simulink model "Switch_block"  (R2021a)
settings: Solver=VariableStepAuto  StartTime=0.0  StopTime=10.0  RelTol=1e-3
settings Model: Creator=HP  LastModifiedBy=HP

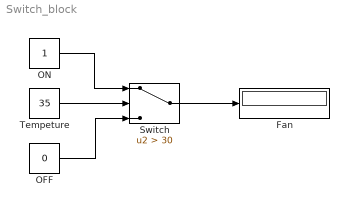
== system Switch_block ==
  Fan : Display
  OFF : Constant  Value=0
  ON : Constant
  Switch : Switch  Criteria=u2 > Threshold  Threshold=30
  Tempeture : Constant  Value=35
  wires:
  Tempeture/1 -> Switch/2
  ON/1 -> Switch/1
  OFF/1 -> Switch/3
  Switch/1 -> Fan/1
